simulink model "SF005A_StOutpCtrl"  (R2013b)
settings: Solver=FixedStepDiscrete  SolverMode=SingleTasking  StartTime=0.0  StopTime=1  FixedStep=0.002  RelTol=1e-3
values from neighbouring files (symbols this model uses):
  ARCHGLBPRM_2MILLISEC_SEC_F32 = DataDict.Constant    [SF005A_StOutpCtrl_DataDict.m]
  ARCHGLBPRM_FLOATZEROTHD_ULS_F32 = DataDict.Constant    [SF005A_StOutpCtrl_DataDict.m]
  BIGSLEW_ULSPERSEC_F32 = DataDict.Constant    [SF005A_StOutpCtrl_DataDict.m]
  DI_CNT_U08 = DataDict.Constant    [SF005A_StOutpCtrl_DataDict.m]
  LOA_CNT_U08 = DataDict.Constant    [SF005A_StOutpCtrl_DataDict.m]
  OPER_CNT_U08 = DataDict.Constant    [SF005A_StOutpCtrl_DataDict.m]
  STRTSTOP_CNT_U08 = DataDict.Constant    [SF005A_StOutpCtrl_DataDict.m]
libraries: NxtrLim x3, simulink x2
(part 2 of 2)

== system SF005A_StOutpCtrl/StOutpCtrl/StOutpCtrlPer1/Target Selection/RateSource/LOA/else ==
  In1 : Inport
  Action Port : ActionPort  ActionType=else
  Out1 : Outport
  wires:
  In1/1 -> Out1/1

== system SF005A_StOutpCtrl/StOutpCtrl/StOutpCtrlPer1/Target Selection/RateSource/Oper/CopyRight2 ==

== system SF005A_StOutpCtrl/StOutpCtrl/StOutpCtrlPer1/Target Selection/RateSource/Oper/If Action Subsystem1 ==
  In1 : Inport
  Action Port : ActionPort  ActionType=then
  Out1 : Outport
  wires:
  In1/1 -> Out1/1

== system SF005A_StOutpCtrl/StOutpCtrl/StOutpCtrlPer1/Target Selection/RateSource/Oper/else ==
  In1 : Inport
  Action Port : ActionPort  ActionType=else
  Out1 : Outport
  wires:
  In1/1 -> Out1/1

== system SF005A_StOutpCtrl/StOutpCtrl/StOutpCtrlPer1/Target Selection/RateSource/StrtStop/CopyRight2 ==

== system SF005A_StOutpCtrl/StOutpCtrl/StOutpCtrlPer1/Target Selection/RateSource/StrtStop/If Action Subsystem1 ==
  In1 : Inport
  Action Port : ActionPort  ActionType=then
  Out1 : Outport
  wires:
  In1/1 -> Out1/1

== system SF005A_StOutpCtrl/StOutpCtrl/StOutpCtrlPer1/Target Selection/RateSource/StrtStop/else ==
  In1 : Inport
  Action Port : ActionPort  ActionType=else
  Out1 : Outport
  wires:
  In1/1 -> Out1/1
